simulink model "deltas"  (R2020a)
settings: Solver=VariableStepAuto  StartTime=0.0  StopTime=10  RelTol=1e-3
values from neighbouring files (symbols this model uses):
  Aa = 2    [dati_tesi_modellosimulink.m]
  g = 9.81    [dati_tesi_modellosimulink.m]
  L = 0.3    [dati_tesi_modellosimulink.m]
  Lc = L/2    (= 0.15)    [dati_tesi_modellosimulink.m]
  M = 4    [dati_tesi_modellosimulink.m]
  mc = 0    [dati_tesi_modellosimulink.m]
  Ra = 1    [dati_tesi_modellosimulink.m]
  wb = 2*pi*2    (= 12.5663706144)    [dati_tesi_modellosimulink.m]
libraries: simulink x9, fuzblock x7, RCTblocks x4, simulink_extras x2
settings Model: Creator=laura  LastModifiedBy=laura

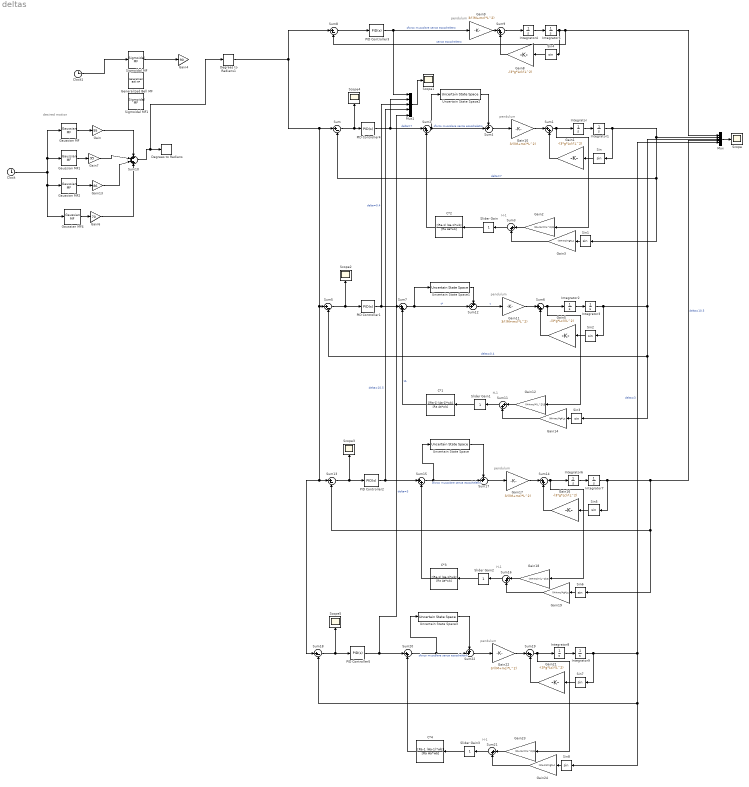
== system deltas ==
  note: H-1
  note: pendulum
  note: pendulum
  note: desired motion
  note: H-1
  note: pendulum
  note: H-1
  note: pendulum
  note: H-1
  note: pendulum
  C*1 : TransferFcn  Numerator=[(Ra-1) (Aa-1)*wb]  Denominator=[Ra Aa*wb]
  C*2 : TransferFcn  Numerator=[(Ra-1) (Aa-1)*wb]  Denominator=[Ra Aa*wb]
  C*3 : TransferFcn  Numerator=[(Ra-1) (Aa-1)*wb]  Denominator=[Ra Aa*wb]
  C*4 : TransferFcn  Numerator=[Ra-1 (Aa-1)*wb]  Denominator=[Ra Aa*wb]
  Clock : Clock
  Clock1 : Clock
  Degrees to Radians : simulink_extras/Transformations/Degrees to Radians
  Degrees to Radians1 : simulink_extras/Transformations/Degrees to Radians
  Gain : Gain  Gain=95
  Gain{1,5,8,16,21} (5 alike) : Gain  Gain=-(3*g*Lc)/(L^2)
  Gain{9..11,17,22} (5 alike) : Gain  Gain=3/((M+mc)*L^2)
  Gain{2,12,18,23} (4 alike) : Gain  Gain=(M+mc)*(L^2)/3
  Gain13 : Gain  Gain=86
  Gain{3,14,19,24} (4 alike) : Gain  Gain=(M+mc)*g*Lc
  Gain4 : Gain  Gain=90
  Gain6 : Gain  Gain=70
  Gain7 : Gain  Gain=95
  Gaussian MF : fuzblock/Membership  Functions/Gaussian MF  sigma=0.4  mu=1.78
      settings: SourceProductBaseCode=FL
  Gaussian MF1 : fuzblock/Membership  Functions/Gaussian MF  sigma=0.4  mu=7
      settings: SourceProductBaseCode=FL
  Gaussian MF2 : fuzblock/Membership  Functions/Gaussian MF  sigma=0.38  mu=3.42
      settings: SourceProductBaseCode=FL
  Gaussian MF4 : fuzblock/Membership  Functions/Gaussian MF  sigma=0.32  mu=2.63
      settings: SourceProductBaseCode=FL
  Generalized Bell MF : fuzblock/Membership  Functions/Generalized Bell MF  a=1.5  b=4  c=6
      settings: SourceProductBaseCode=FL
  Integrator{,1..9} (10 alike) : Integrator
  Mux : Mux  Inputs=5
  Mux1 : Mux  Inputs=5
  PID Controller{1..5} (5 alike) : simulink/Continuous/PID Controller  Controller=PID  Form=Parallel  TimeDomain=Continuous-time  UseExternalTs=off  SampleTime=-1  IntegratorMethod=Forward Euler  FilterMethod=Forward Euler  ControllerParametersSource=internal  P=20.396  I=105.7651  D=6.3413  UseFilter=on  N=150.7964  TunerSelectOption=Transfer Function Based (PID Tuner App)  InitialConditionSource=internal  InitialConditionForIntegrator=0  InitialConditionForFilter=0  DifferentiatorICPrevScaledInput=0  ExternalReset=none  TrackingMode=off  Kt=1  LimitOutput=off  UpperSaturationLimit=inf  LowerSaturationLimit=-inf  LinearizeAsGain=on  AntiWindupMode=none  Kb=1  POutMin=[]  POutMax=[]  IOutMin=[]  IOutMax=[]  DOutMin=[]  DOutMax=[]  NOutMin=[]  NOutMax=[]  SumOutMin=[]  SumOutMax=[]  SaturationOutMin=[]  SaturationOutMax=[]  PParamMin=[]  PParamMax=[]  IParamMin=[]  IParamMax=[]  DParamMin=[]  DParamMax=[]  NParamMin=[]  NParamMax=[]  KbParamMin=[]  KbParamMax=[]  KtParamMin=[]  KtParamMax=[]  KbOutMin=[]  KbOutMax=[]  KtOutMin=[]  KtOutMax=[]  IntegratorOutMin=[]  IntegratorOutMax=[]  FilterOutMin=[]  FilterOutMax=[]  SumI1OutMin=[]  SumI1OutMax=[]  SumI2OutMin=[]  SumI2OutMax=[]  SumI3OutMin=[]  SumI3OutMax=[]  SumI4OutMin=[]  SumI4OutMax=[]  SumDOutMin=[]  SumDOutMax=[]  DifferentiatorOutMin=[]  DifferentiatorOutMax=[]  FilterDiffOutCoefMin=[]  FilterDiffOutCoefMax=[]  ReciprocalOutMin=[]  ReciprocalOutMax=[]  SumDenOutMin=[]  SumDenOutMax=[]  SumNumOutMin=[]  SumNumOutMax=[]  DivideOutMin=[]  DivideOutMax=[]  UdiffTsProdOutMin=[]  UdiffTsProdOutMax=[]  NTsProdOutMin=[]  NTsProdOutMax=[]  UintegralTsProdOutMin=[]  UintegralTsProdOutMax=[]  UngainTsProdOutMin=[]  UngainTsProdOutMax=[]  IntegratorContinuousStateAttributes=''  IntegratorStateMustResolveToSignalObject=off  IntegratorRTWStateStorageClass=Auto  FilterContinuousStateAttributes=''  FilterStateMustResolveToSignalObject=off  FilterRTWStateStorageClass=Auto  ParallelPVariant=InternalParameters  IdealPVariant=Disabled  IVariant=InternalParameters  DVariant=InternalParameters  IntegratorVariant=Continuous  SatVariant=Disabled  AWVariant=Passthrough  PCopyVariant=Disabled  TRVariant=Disabled  FdbkBlocksVariant=Forward  IdealPFdbkVariant=Disabled  SatFdbkVariant=Disabled  DerivativeFilterVariant=ContFilter  NVariant=InternalParameters  NCopyVariant=Disabled  FilterICVariant=InternalICsFilter  IntegratorICVariant=InternalICs  ExternalResetVariant=Disabled  TRSumVariant=Passthrough  SumFdbkVariant=Disabled  SumVariant=Sum_PID  TsampFilterVariant=InternalTs  TsampNgainVariant=Passthrough  TsampIntegralVariant=Passthrough
  Scope{,1..5} (6 alike) : Scope
  Sigmoidal MF : fuzblock/Membership  Functions/Sigmoidal MF  a=4  c=5
      settings: SourceProductBaseCode=FL
  Sigmoidal MF1 : fuzblock/Membership  Functions/Sigmoidal MF  a=-4  c=5
      settings: SourceProductBaseCode=FL
  Sin{,1..8} (9 alike) : Trigonometry
  Slider Gain{,1..3} (4 alike) : simulink/Math Operations/Slider Gain  gain=1  low=0  high=2
  Sum{,5,8,13,18} (5 alike) : Sum  Inputs=|+-
  Sum{1..3,6..7,9,11,14..16,19..21} (13 alike) : Sum  Inputs=|++
  Sum10 : Sum  Inputs=++++
  Sum{4,12,17,22} (4 alike) : Sum  Inputs=++|
  Uncertain State Space : RCTblocks/Uncertain State Space  Tag=USS  USystem=delta_sample2  UValue=[]  X0=[]  uX0=[]
      settings: SourceProductBaseCode=RC
  Uncertain State Space1 : RCTblocks/Uncertain State Space  Tag=USS  USystem=delta_sample1  UValue=[]  X0=[]  uX0=[]
      settings: SourceProductBaseCode=RC
  Uncertain State Space2 : RCTblocks/Uncertain State Space  Tag=USS  USystem=delta_sample  UValue=[]  X0=[]  uX0=[]
      settings: SourceProductBaseCode=RC
  Uncertain State Space3 : RCTblocks/Uncertain State Space  Tag=USS  USystem=delta_sample3  UValue=[]  X0=[]  uX0=[]
      settings: SourceProductBaseCode=RC
  wires:
  Sum/1 -> PID Controller4/1, Scope4/1
  Sin1/1 -> Gain3/1
  Gain10/1 -> Sum1/1
  Integrator4/1 -> Integrator5/1
  Sum3/1 -> Slider Gain/1
  Sin4/1 -> Gain8/1
  Gain9/1 -> Sum9/1
  Mux1/1 -> Scope1/1
  Sum9/1 -> Integrator4/1
  Gain8/1 -> Sum9/2
  PID Controller4/1 -> Mux1/2, Sum2/1  "delta=7"
  Sin/1 -> Gain1/1
  Gain1/1 -> Sum1/2
  PID Controller3/1 -> Gain9/1, Mux1/1  "sforzo muscolare senza esoscheletro"
  C*2/1 -> Sum2/2
  Integrator5/1 -> Mux/1, Sum8/2, Sin4/1  "senza esoscheletro"
  Sum1/1 -> Integrator/1, Gain2/1
  Gain3/1 -> Sum3/2
  Gain2/1 -> Sum3/1
  Sum8/1 -> PID Controller3/1
  Integrator1/1 -> Sin/1, Sin1/1, Sum/2, Mux/2  "delta=7"
  Integrator/1 -> Integrator1/1
  Mux/1 -> Scope/1
  Gain7/1 -> Sum10/2
  Gain13/1 -> Sum10/3
  Clock/1 -> Gaussian MF/1, Gaussian MF1/1, Gaussian MF4/1, Gaussian MF2/1
  Gain/1 -> Sum10/1
  Gaussian MF1/1 -> Gain7/1
  Gaussian MF2/1 -> Gain13/1
  Gain6/1 -> Sum10/4
  Sum10/1 -> Degrees to Radians1/1, Degrees to Radians/1
  Gaussian MF/1 -> Gain/1
  Gaussian MF4/1 -> Gain6/1
  Uncertain State Space2/1 -> Sum4/1
  Sum2/1 -> Uncertain State Space2/1, Sum4/2  "sforzo muscolare senza esoscheletro"
  Sum4/1 -> Gain10/1
  Slider Gain/1 -> C*2/1
  Uncertain State Space1/1 -> Sum12/1
  Sum7/1 -> Uncertain State Space1/1, Sum12/2  "t*"
  Sin2/1 -> Gain5/1
  Sum6/1 -> Integrator2/1, Gain12/1
  Gain12/1 -> Sum11/1
  C*1/1 -> Sum7/2  "tA"
  Gain14/1 -> Sum11/2
  PID Controller1/1 -> Mux1/3, Sum7/1  "delta=0.4"
  Integrator2/1 -> Integrator3/1
  Integrator3/1 -> Sin2/1, Sin3/1, Sum5/2, Mux/3  "delta=0.4"
  Sin3/1 -> Gain14/1
  Sum12/1 -> Gain11/1  "t"
  Gain11/1 -> Sum6/1
  Sum11/1 -> Slider Gain1/1
  Sum5/1 -> PID Controller1/1, Scope2/1
  Slider Gain1/1 -> C*1/1
  Gain5/1 -> Sum6/2
  Uncertain State Space/1 -> Sum17/1
  Sum15/1 -> Sum17/2, Uncertain State Space/1  "sforzo muscolare senza esoscheletro"
  Sin5/1 -> Gain16/1
  Sum14/1 -> Integrator6/1, Gain18/1
  Gain18/1 -> Sum16/1
  C*3/1 -> Sum15/2
  Gain19/1 -> Sum16/2
  PID Controller2/1 -> Mux1/4, Sum15/1  "delta=10.5"
  Integrator6/1 -> Integrator7/1
  Integrator7/1 -> Sin5/1, Mux/4, Sin6/1, Sum13/2  "delta=10.5"
  Sin6/1 -> Gain19/1
  Sum17/1 -> Gain17/1
  Gain17/1 -> Sum14/1
  Sum16/1 -> Slider Gain2/1
  Sum13/1 -> PID Controller2/1, Scope3/1
  Slider Gain2/1 -> C*3/1
  Gain16/1 -> Sum14/2
  Uncertain State Space3/1 -> Sum22/1
  Sum20/1 -> Uncertain State Space3/1, Sum22/2  "sforzo muscolare senza esoscheletro"
  Sin7/1 -> Gain21/1
  Sum19/1 -> Integrator8/1, Gain23/1
  Gain23/1 -> Sum21/1
  C*4/1 -> Sum20/2
  Gain24/1 -> Sum21/2
  PID Controller5/1 -> Mux1/5, Sum20/1  "delta=3"
  Integrator8/1 -> Integrator9/1
  Integrator9/1 -> Sin7/1, Sin8/1, Sum18/2, Mux/5  "delta=3"
  Sin8/1 -> Gain24/1
  Sum22/1 -> Gain22/1
  Gain22/1 -> Sum19/1
  Sum21/1 -> Slider Gain3/1
  Sum18/1 -> PID Controller5/1, Scope5/1
  Slider Gain3/1 -> C*4/1
  Gain21/1 -> Sum19/2
  Clock1/1 -> Sigmoidal MF/1
  Sigmoidal MF/1 -> Gain4/1
  Degrees to Radians1/1 -> Sum18/1, Sum13/1, Sum5/1, Sum/1, Sum8/1
